simulink model "myModel_discrete"  (R2023b)
settings: Solver=VariableStepAuto  StartTime=0.0  StopTime=10  RelTol=1e-3
values from neighbouring files (symbols this model uses):
  A = [0, 0               ,   1           , 0 ... (first row only)    [mytask.m]
  B = [0, 0,  1/mc,   1/(L*mc)]'    [mytask.m]
  C = [1, 0,  0,  0]    [mytask.m]
  K_d = acker(Ad,Bd,des_poles_d)    [mytask.m]
  K_lqr = lqr(A,B,Q,R)    [mytask.m]
  Ts = 0.1    [mytask.m]
  x0 = [0;    5*pi/180;   0;  0]    [mytask.m]
settings Model: Creator=admin  LastModifiedBy=admin

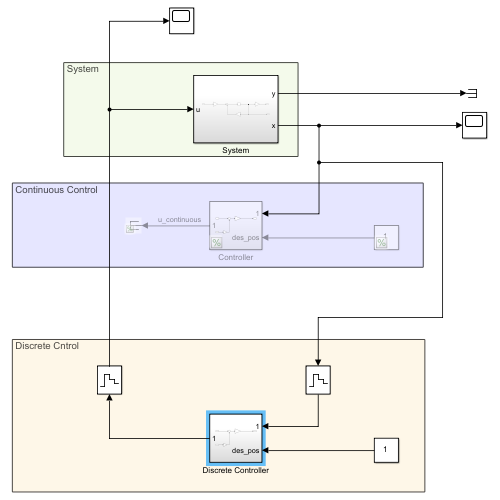
[thumbnail: Simulink's stored preview of the top-level diagram]
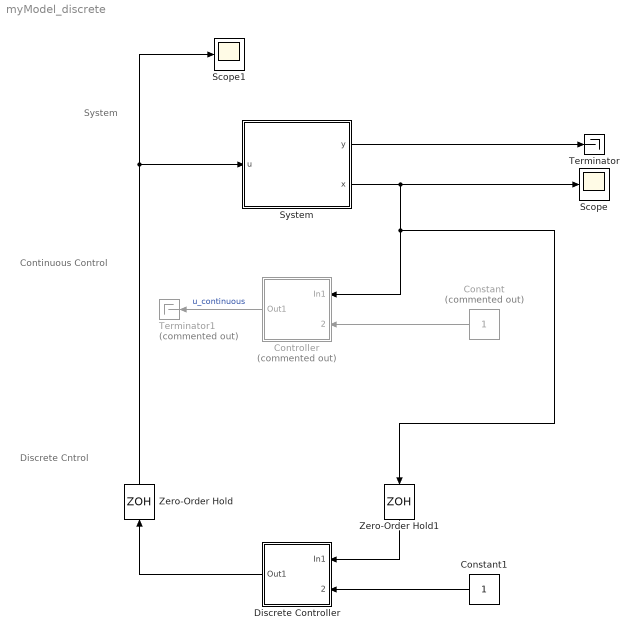
== system myModel_discrete ==
  note: System
  note: Discrete Cntrol
  note: Continuous Control
  Constant : Constant  Commented=on
  Constant1 : Constant
  Controller : Subsystem  Commented=on
  Discrete Controller : Subsystem
  Scope : Scope
  Scope1 : Scope
  System : Subsystem
  Terminator : Terminator
  Terminator1 : Terminator  Commented=on
  Zero-Order Hold : ZeroOrderHold  SampleTime=Ts
  Zero-Order Hold1 : ZeroOrderHold  SampleTime=Ts
  wires:
  System/1(y) -> Terminator/1
  System/2(x) -> Controller/1(In1), Zero-Order Hold1/1, Scope/1
  Constant/1 -> Controller/2(des_pos)
  Controller/1(Out1) -> Terminator1/1  "u_continuous"
  Zero-Order Hold1/1 -> Discrete Controller/1(In1)
  Constant1/1 -> Discrete Controller/2(des_pos)
  Discrete Controller/1(Out1) -> Zero-Order Hold/1
  Zero-Order Hold/1 -> System/1(u), Scope1/1

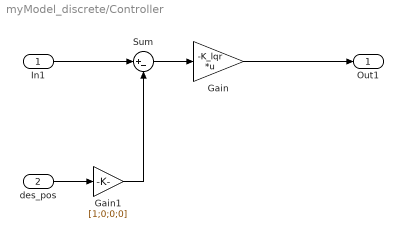
== system myModel_discrete/Controller ==
  In1 : Inport
  des_pos : Inport  Port=2
  Gain : Gain  Gain=-K_lqr  Multiplication=Matrix(K*u)
  Gain1 : Gain  Gain=[1;0;0;0]
  Sum : Sum  Inputs=|+-
  Out1 : Outport
  wires:
  Gain/1 -> Out1/1
  Sum/1 -> Gain/1
  In1/1 -> Sum/1
  des_pos/1 -> Gain1/1
  Gain1/1 -> Sum/2

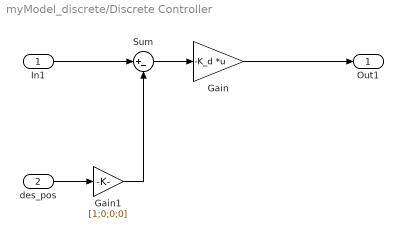
== system myModel_discrete/Discrete Controller ==
  In1 : Inport
  des_pos : Inport  Port=2
  Gain : Gain  Gain=-K_d  Multiplication=Matrix(K*u)
  Gain1 : Gain  Gain=[1;0;0;0]
  Sum : Sum  Inputs=|+-
  Out1 : Outport
  wires:
  Gain/1 -> Out1/1
  Sum/1 -> Gain/1
  In1/1 -> Sum/1
  des_pos/1 -> Gain1/1
  Gain1/1 -> Sum/2

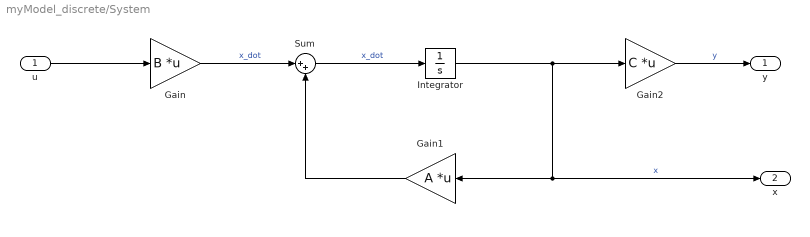
== system myModel_discrete/System ==
  u : Inport
  Gain : Gain  Gain=B  Multiplication=Matrix(K*u)
  Gain1 : Gain  Gain=A  Multiplication=Matrix(K*u)
  Gain2 : Gain  Gain=C  Multiplication=Matrix(K*u)
  Integrator : Integrator  InitialCondition=x0
  Sum : Sum  Inputs=|++
  y : Outport
  x : Outport  Port=2
  wires:
  Gain/1 -> Sum/1  "x_dot"
  Gain2/1 -> y/1  "y"
  Sum/1 -> Integrator/1  "x_dot"
  Gain1/1 -> Sum/2
  Integrator/1 -> x/1, Gain1/1, Gain2/1  "x"
  u/1 -> Gain/1
